simulink model "sl_ibvs"  (Simulink 8.0)
settings: Solver=ode45  StartTime=0.0  StopTime=10  RelTol=1e-3
InitFcn:
  | cam = CentralCamera('default')
undefined symbols (not defined in the file or in its folder): mkgrid, transl, trotz
libraries: roblocks x4
settings Model: Creator=pic  LastModifiedBy=corkep  ExtModeTrigMode=oneshot  ExtModeArmWhenConnect=off
settings DataIOCC: LimitDataPoints=off  SaveFormat=Structure  SignalLoggingSaveFormat=ModelDataLogs  ReturnWorkspaceOutputs=on
settings OptimizationCC: BlockReduction=off  BooleanDataType=off  InitFltsAndDblsToZero=on
settings DebuggingCC: SaveWithParameterizedLinksMsg=none  SignalResolutionControl=TryResolveAllWithWarning  SolverPrmCheckMsg=none  MultiTaskDSMMsg=warning  MultiTaskCondExecSysMsg=none  FcnCallInpInsideContextMsg=UseLocalSettings  StrictBusMsg=None
settings HardwareCC: TargetUnknown=on
settings RTWCC: IncludeERTFirstTime=on
settings GRTTargetCC: ModelReferenceCompliant=off  CompOptLevelCompliant=off  CombineOutputUpdateFcns=off  MatFileLogging=off  GRTInterface=on

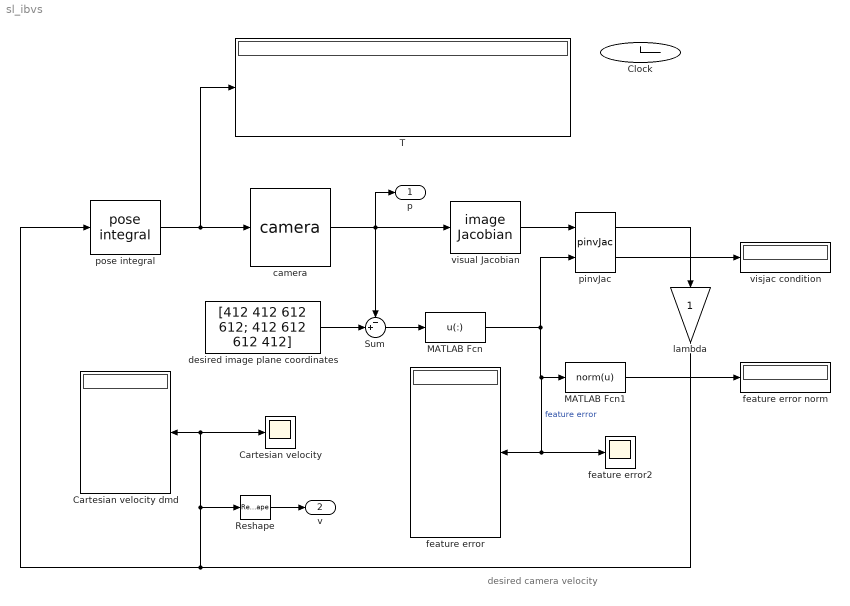
== system sl_ibvs ==
  note: desired camera velocity
  Cartesian velocity : Scope
      settings: TimeRange=10  YMin=-3  YMax=0.75
  Cartesian velocity dmd : Display
      settings: Format=bank
  Clock : Clock
  MATLAB Fcn : MATLABFcn  MATLABFcn=u(:)  Output1D=off
  MATLAB Fcn1 : MATLABFcn  MATLABFcn=norm(u)
  Reshape : Reshape  OutputDimensionality=Customize  OutputDimensions=6
  Sum : Sum  Inputs=-+|  SaturateOnIntegerOverflow=on  InputSameDT=on  OutDataTypeStr=Inherit: Same as first input
  T : Display
  camera : roblocks/Vision/camera  cam=cam  points=mkgrid(2, 0.5, transl(0,0,3))
  desired image plane coordinates : Constant  Value=[412 412 612 612; 412 612 612 412]  VectorParams1D=off
  feature error : Display
      settings: Format=bank
  feature error norm : Display
  feature error2 : Scope
      settings: TimeRange=20  YMin=-150  YMax=150
  lambda : Gain  SaturateOnIntegerOverflow=on  OutDataTypeStr=Inherit: Same as input  ParamDataTypeStr=Inherit: Same as input
  pinvJac : roblocks/Vision/pinvJac
  pose integral : roblocks/Kinematics/pose integral  T0=transl(0,0,1)*trotz(1.5)  dt=0.02
  visjac condition : Display
  visual Jacobian : roblocks/Vision/image Jacobian  cam=cam  z=3
  p : Outport
  v : Outport  Port=2
  wires:
  camera/1 -> Sum/1, visual Jacobian/1, p/1
  Sum/1 -> MATLAB Fcn/1
  desired image plane coordinates/1 -> Sum/2
  MATLAB Fcn/1 -> MATLAB Fcn1/1, feature error2/1, feature error/1, pinvJac/2  "feature error"
  pinvJac/2 -> visjac condition/1
  MATLAB Fcn1/1 -> feature error norm/1
  pinvJac/1 -> lambda/1
  pose integral/1 -> T/1, camera/1
  visual Jacobian/1 -> pinvJac/1
  lambda/1 -> Cartesian velocity dmd/1, Cartesian velocity/1, Reshape/1, pose integral/1
  Reshape/1 -> v/1
